simulink model "untitled"  (R2025b)
settings: Solver=VariableStepAuto  StartTime=0.0  StopTime=67.0  RelTol=1e-3
settings Model: Creator=User  LastModifiedBy=User

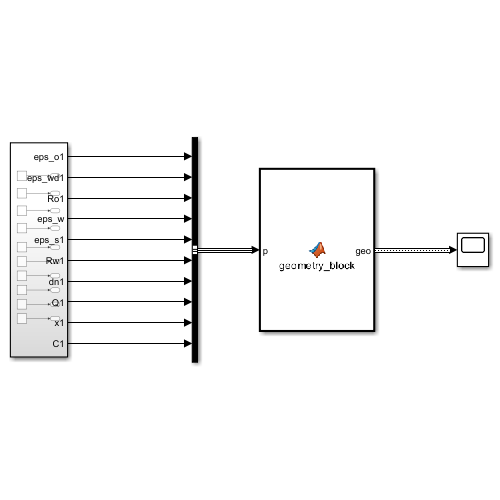
[thumbnail: Simulink's stored preview of the top-level diagram]
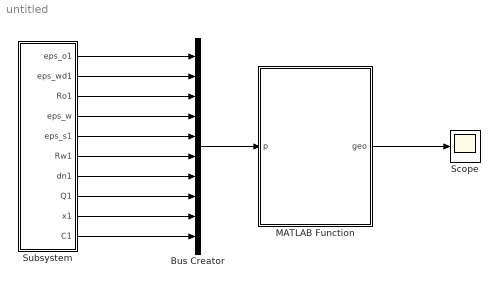
== system untitled ==
  Bus Creator : BusCreator  Inputs=10  OutDataTypeStr=Bus: BusTricInputs
  MATLAB Function : MATLAB Function  TreatAsAtomicUnit=on
  Scope : Scope
      settings: ActiveDisplayYMinimum=-0.21112892830066032  ActiveDisplayYMaximum=2.6538939689506353
  Subsystem : Subsystem
  wires:
  MATLAB Function/1(geo) -> Scope/1
  Bus Creator/1 -> MATLAB Function/1(p)
  Subsystem/1(eps_o1) -> Bus Creator/1
  Subsystem/2(eps_wd1) -> Bus Creator/2
  Subsystem/3(Ro1) -> Bus Creator/3
  Subsystem/4(eps_w) -> Bus Creator/4
  Subsystem/5(eps_s1) -> Bus Creator/5
  Subsystem/6(Rw1) -> Bus Creator/6
  Subsystem/7(dn1) -> Bus Creator/7
  Subsystem/8(Q1) -> Bus Creator/8
  Subsystem/9(x1) -> Bus Creator/9
  Subsystem/10(C1) -> Bus Creator/10

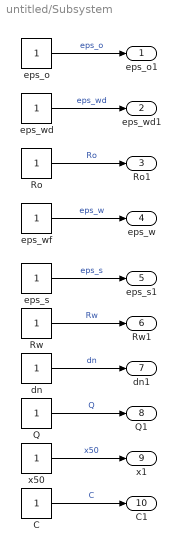
== system untitled/Subsystem ==
  C : Constant
  Q : Constant
  Ro : Constant
  Rw : Constant
  dn : Constant
  eps_o : Constant
  eps_s : Constant
  eps_wd : Constant
  eps_wf : Constant
  x50 : Constant
  eps_o1 : Outport
  eps_wd1 : Outport  Port=2
  Ro1 : Outport  Port=3
  eps_w : Outport  Port=4
  eps_s1 : Outport  Port=5
  Rw1 : Outport  Port=6
  dn1 : Outport  Port=7
  Q1 : Outport  Port=8
  x1 : Outport  Port=9
  C1 : Outport  Port=10
  wires:
  eps_o/1 -> eps_o1/1  "eps_o"
  eps_wd/1 -> eps_wd1/1  "eps_wd"
  C/1 -> C1/1  "C"
  eps_wf/1 -> eps_w/1  "eps_w"
  Q/1 -> Q1/1  "Q"
  Rw/1 -> Rw1/1  "Rw"
  Ro/1 -> Ro1/1  "Ro"
  eps_s/1 -> eps_s1/1  "eps_s"
  dn/1 -> dn1/1  "dn"
  x50/1 -> x1/1  "x50"

== matlab function untitled/MATLAB Function ==
  data: geo output Bus: BusTricGeo; p input size=1; TricParams parameter
function geo = geometry_block(p, TricParams)
pc = TricParams;
%#codegen
% p  — варьируемые параметры (Bus): Q, dn, Ro, Rw, eps_o, eps_wd, eps_w, eps_s
% pc — стационарные параметры (Parameter): Rd, Wsc, Lpond, alpha, Lsep,
%      mu_s, phi_sed, u_conv, rho_s, rho_w, rho_o, eta_w, eta_o, C, n

G = 9.81;

% --- вращение и геометрия шнека ---
omega = sqrt(p.C * G / pc.Rd);
beta  = atan2(pc.Wsc, 2*pi*pc.Rd);

% --- осевая длина ячейки ---
Lax = pc.Lpond / pc.n;

% --- вклад конуса в осветление ---
t = tan(pc.alpha * pi/180);
L_cone = (pc.Rd^3 - p.Rw^3) / (3*t) / pc.Rd^2;

if pc.Lsep > 0
    L_eff = pc.Lsep;
else
    L_eff = pc.Lpond + L_cone;
end
f_clar = L_eff / pc.Lpond;

% --- осевая скорость выноса кека ---
kappa = atan(pc.mu_s) + beta;
eff   = 1 / (1 + tan(beta)*tan(kappa));
u_ax  = pc.Wsc * p.dn/60 * eff * pc.u_conv;

% --- есть ли нефтяная фаза ---
has_oil = (p.eps_o + p.eps_wd) > 0;

% --- граница нефть-вода из баланса давлений ---
if has_oil
    r2 = (pc.rho_w*p.Rw^2 - pc.rho_o*p.Ro^2) / (pc.rho_w - pc.rho_o);
    r_i = sqrt(max(r2, 0));
    r_i = min(max(r_i, p.Ro), pc.Rd);   % clip как в Python
else
    r_i = p.Rw;
end

% --- расходы по кольцам ---
Qo = p.Q * (p.eps_o + p.eps_wd);
Qw = p.Q * (p.eps_w + p.eps_s);

% --- сборка выходной шины ---
geo.omega   = omega;
geo.beta    = beta;
geo.Lax     = Lax;
geo.L_cone  = L_cone;
geo.f_clar  = f_clar;
geo.u_ax    = u_ax;
geo.has_oil = has_oil;
geo.r_i     = r_i;
geo.Qo      = Qo;
geo.Qw      = Qw;
